simulink model "Sim_dyn_base"  (R2018b)
settings: Solver=VariableStepAuto  StartTime=0.0  StopTime=inf  RelTol=1e-3
values from neighbouring files (symbols this model uses):
  q_0 = zeros(5,1).'    [DATAsim.m]
undefined symbols (not defined in the file or in its folder): limit_check, v_max
libraries: simulink x1
settings Model: Creator=Francesco Gennari  LastModifiedBy=Francesco Gennari
settings DebuggingCC: UnderSpecifiedDimensionMsg=warning

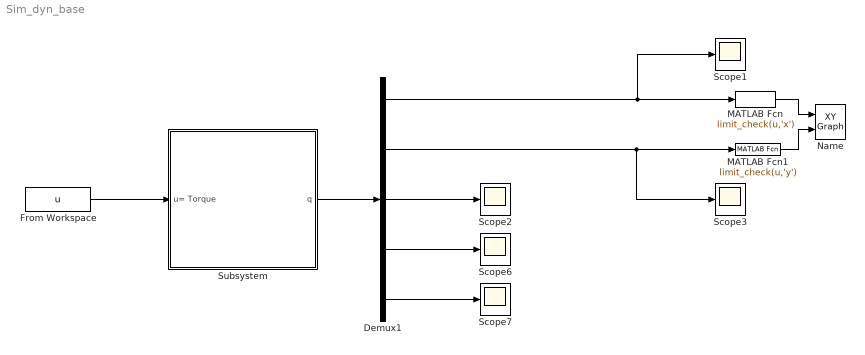
== system Sim_dyn_base ==
  Demux1 : Demux  Outputs=[1 1 1 1 1]
  From Workspace : FromWorkspace  VariableName=u
  MATLAB Fcn : MATLABFcn  MATLABFcn=limit_check(u,'x')
  MATLAB Fcn1 : MATLABFcn  MATLABFcn=limit_check(u,'y')
  Name : simulink/Sinks/XY Graph  xmin=-14.8999  xmax=77.9146  ymin=-49.5507  ymax=15.0072  st=-1
  Scope{1..3,6..7} (5 alike) : Scope
  Subsystem : Subsystem
  wires:
  Subsystem/1(q) -> Demux1/1
  Demux1/1 -> Scope1/1, MATLAB Fcn/1
  Demux1/2 -> MATLAB Fcn1/1, Scope3/1
  Demux1/3 -> Scope2/1
  MATLAB Fcn1/1 -> Name/2
  MATLAB Fcn/1 -> Name/1
  Demux1/4 -> Scope6/1
  Demux1/5 -> Scope7/1
  From Workspace/1 -> Subsystem/1(u= Torque)

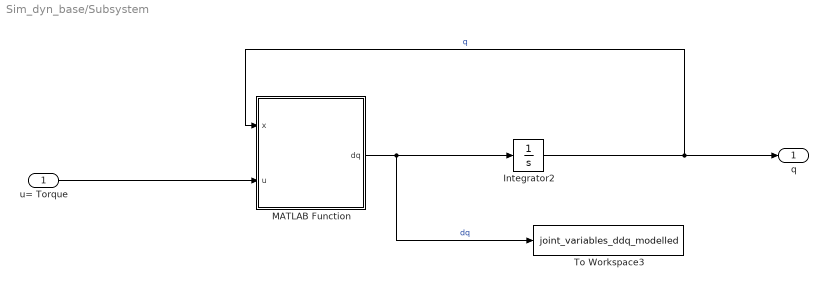
== system Sim_dyn_base/Subsystem ==
  u= Torque : Inport
  Integrator2 : Integrator  InitialCondition=[q_0]  UpperSaturationLimit=v_max  LowerSaturationLimit=-v_max  ContinuousStateAttributes='velocity'
  MATLAB Function : MATLAB Function  TreatAsAtomicUnit=on
  To Workspace3 : ToWorkspace  VariableName=joint_variables_ddq_modelled  SaveFormat=Timeseries  SampleTime=-1
  q : Outport
  wires:
  Integrator2/1 -> q/1, MATLAB Function/1(x)  "q"
  MATLAB Function/1(dq) -> Integrator2/1, To Workspace3/1  "dq"
  u= Torque/1 -> MATLAB Function/2(u)

== matlab function Sim_dyn_base/Subsystem/MATLAB Function ==
  data: x input; dq output; u input
function dq   = sys_dynamics(x,u)

[A,F,D] = matriceseval(x);
 
dq=A*x+F*u+D;


end
